simulink model "Motor_Pos"  (R2017a)
settings: Solver=ode45  StartTime=0.0  StopTime=10.0  RelTol=1e-3
undefined symbols (not defined in the file): b, J, K, L, R
settings Model: Creator=sansh  LastModifiedBy=judson3

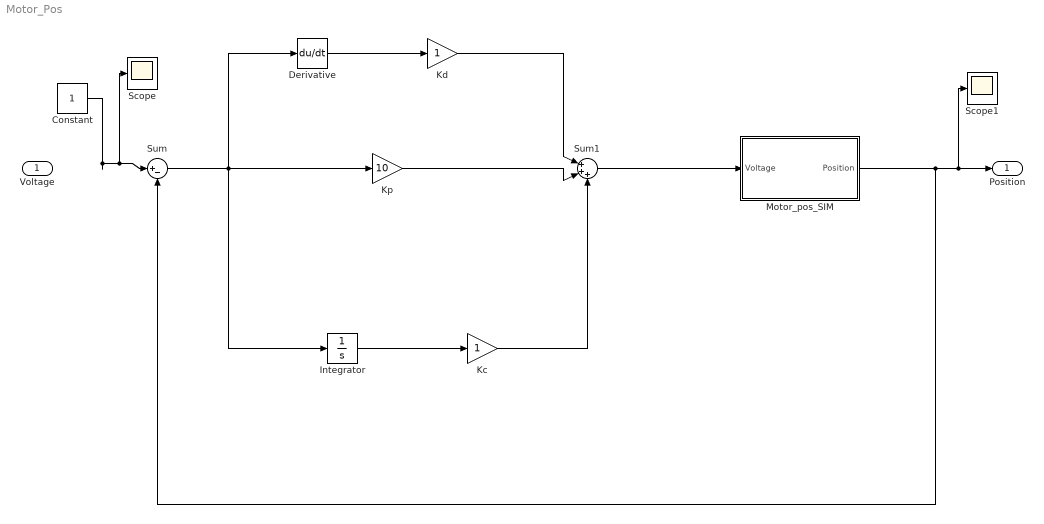
== system Motor_Pos ==
  Voltage : Inport
  Constant : Constant
  Derivative : Derivative
  Integrator : Integrator
  Kc : Gain
  Kd : Gain
  Kp : Gain  Gain=10
  Motor_pos_SIM : Subsystem
  Scope : Scope
  Scope1 : Scope
  Sum : Sum  Inputs=|+-
  Sum1 : Sum  Inputs=|+++
  Position : Outport
  wires:
  Motor_pos_SIM/1(Position) -> Sum/2, Scope1/1, Position/1
  Sum1/1 -> Motor_pos_SIM/1(Voltage)
  Sum/1 -> Integrator/1, Derivative/1, Kp/1
  Kp/1 -> Sum1/2
  Derivative/1 -> Kd/1
  Kd/1 -> Sum1/1
  Integrator/1 -> Kc/1
  Kc/1 -> Sum1/3
  Constant/1 -> Scope/1, Sum/1

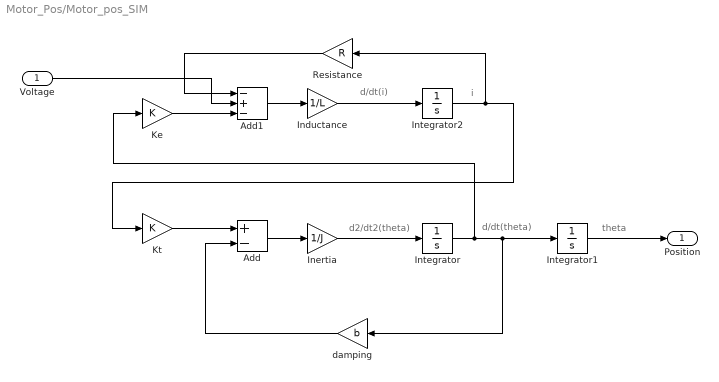
== system Motor_Pos/Motor_pos_SIM ==
  note: i
  note: d/dt(i)
  note: d2/dt2(theta)
  note: d/dt(theta)
  note: theta
  Voltage : Inport
  Add : Sum  Inputs=+-
  Add1 : Sum  Inputs=-+-
  Inductance : Gain  Gain=1/L
  Inertia : Gain  Gain=1/J
  Integrator : Integrator
  Integrator1 : Integrator
  Integrator2 : Integrator
  Ke : Gain  Gain=K
  Kt : Gain  Gain=K
  Resistance : Gain  Gain=R
  damping : Gain  Gain=b
  Position : Outport
  wires:
  Inertia/1 -> Integrator/1
  Inductance/1 -> Integrator2/1
  Integrator2/1 -> Resistance/1, Kt/1
  Integrator/1 -> Ke/1, damping/1, Integrator1/1
  Integrator1/1 -> Position/1
  Voltage/1 -> Add1/2
  Add/1 -> Inertia/1
  damping/1 -> Add/2
  Kt/1 -> Add/1
  Resistance/1 -> Add1/1
  Ke/1 -> Add1/3
  Add1/1 -> Inductance/1
